simulink model "fullact_invpend647"  (Simulink 7.6)
settings: Solver=ode45  StartTime=0.0  StopTime=10  FixedStep=Ts  RelTol=1e-5
values from neighbouring files (symbols this model uses):
  A1 = 0.1    [setup647.m]
  A2 = 0.25    [setup647.m]
  w1 = 2    [setup647.m]
  w2 = 3    [setup647.m]
  Z0 = [0;pi/4;0;0]    [setup647.m]
undefined symbols (not defined in the file or in its folder): invdyn647, stateder_invpend647
settings Model: Creator=rhanz  LastModifiedBy=rhanz
settings DataIOCC: SignalLogging=off  Refine=2
settings DebuggingCC: FcnCallInpInsideContextMsg=Enable All

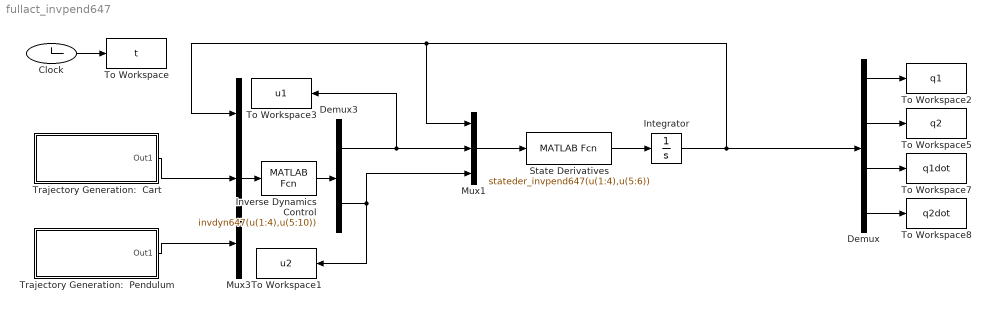
== system fullact_invpend647 ==
  Clock : Clock
      settings: Decimation=10
  Demux : Demux
  Demux3 : Demux  Outputs=2
  Integrator : Integrator  InitialCondition=Z0
  Inverse Dynamics Control : MATLABFcn  MATLABFcn=invdyn647(u(1:4),u(5:10))  OutputDimensions=2
  Mux1 : Mux  Inputs=3
  Mux3 : Mux  Inputs=3
  State Derivatives : MATLABFcn  MATLABFcn=stateder_invpend647(u(1:4),u(5:6))  OutputDimensions=4  Output1D=off
  To Workspace : ToWorkspace  VariableName=t  SampleTime=-1  SaveFormat=Array
  To Workspace1 : ToWorkspace  VariableName=u2  SampleTime=-1  SaveFormat=Array
  To Workspace2 : ToWorkspace  VariableName=q1  SampleTime=-1  SaveFormat=Array
  To Workspace3 : ToWorkspace  VariableName=u1  SampleTime=-1  SaveFormat=Array
  To Workspace5 : ToWorkspace  VariableName=q2  SampleTime=-1  SaveFormat=Array
  To Workspace7 : ToWorkspace  VariableName=q1dot  SampleTime=-1  SaveFormat=Array
  To Workspace8 : ToWorkspace  VariableName=q2dot  SampleTime=-1  SaveFormat=Array
  Trajectory Generation:  Cart : Subsystem
  Trajectory Generation:  Pendulum : Subsystem
  wires:
  Clock/1 -> To Workspace/1
  Demux/1 -> To Workspace2/1
  Demux/2 -> To Workspace5/1
  Trajectory Generation:  Cart/1(Out1) -> Mux3/2
  Trajectory Generation:  Pendulum/1(Out1) -> Mux3/3
  Mux3/1 -> Inverse Dynamics Control/1
  Inverse Dynamics Control/1 -> Demux3/1
  Mux1/1 -> State Derivatives/1
  State Derivatives/1 -> Integrator/1
  Demux/3 -> To Workspace7/1
  Demux/4 -> To Workspace8/1
  Integrator/1 -> Demux/1, Mux3/1, Mux1/1
  Demux3/2 -> To Workspace1/1, Mux1/3
  Demux3/1 -> Mux1/2, To Workspace3/1

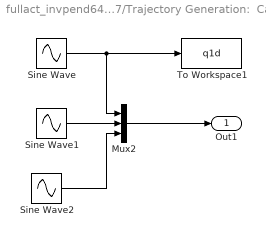
== system fullact_invpend647/Trajectory Generation:  Cart ==
  Mux2 : Mux  Inputs=3
  Sine Wave : Sin  Amplitude=A1  Frequency=w1  SampleTime=0
  Sine Wave1 : Sin  Amplitude=A1*w1  Frequency=w1  Phase=pi/2  SampleTime=0
  Sine Wave2 : Sin  Amplitude=A1*w1^2  Frequency=w1  Phase=pi  SampleTime=0
  To Workspace1 : ToWorkspace  VariableName=q1d  SampleTime=-1  SaveFormat=Array
  Out1 : Outport
  wires:
  Sine Wave/1 -> Mux2/1, To Workspace1/1
  Mux2/1 -> Out1/1
  Sine Wave2/1 -> Mux2/3
  Sine Wave1/1 -> Mux2/2

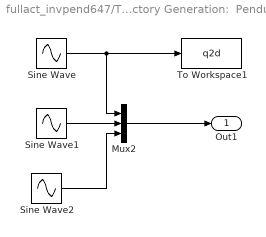
== system fullact_invpend647/Trajectory Generation:  Pendulum ==
  Mux2 : Mux  Inputs=3
  Sine Wave : Sin  Amplitude=A2  Frequency=w2  SampleTime=0
  Sine Wave1 : Sin  Amplitude=A2*w2  Frequency=w2  Phase=pi/2  SampleTime=0
  Sine Wave2 : Sin  Amplitude=A2*w2^2  Frequency=w2  Phase=pi  SampleTime=0
  To Workspace1 : ToWorkspace  VariableName=q2d  SampleTime=-1  SaveFormat=Array
  Out1 : Outport
  wires:
  Sine Wave1/1 -> Mux2/2
  Sine Wave2/1 -> Mux2/3
  Mux2/1 -> Out1/1
  Sine Wave/1 -> To Workspace1/1, Mux2/1
